simulink model "VAS_exec"  (Simulink 3.00)
undefined symbols (not defined in the file): BETA, PROJECT, REXYGEN, RPi, VAS, W1_owscfg
libraries: execlib x12

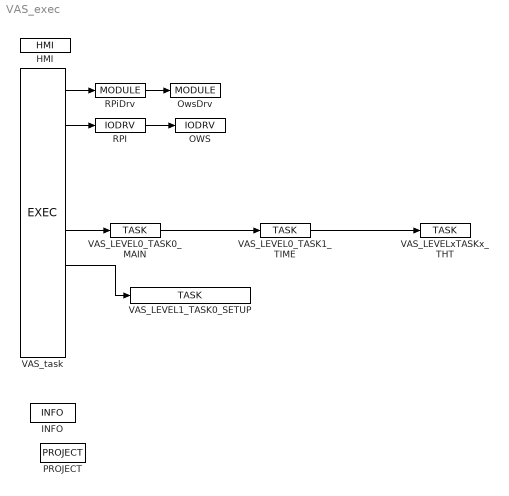
== system VAS_exec ==
  HMI : execlib/HMI  IncludeHMI=on  HmiDir=hmi  SourceDir=hmisrc  GenerateWebWatch=off  GenerateRexHMI=on  RedirectToHMI=on  Compression=on
  INFO : execlib/INFO  Title=VAS-REXYGEN-PROJECT-BETA  Author=Christopher Rothfeldt  Description=Vivarium Automation Server developed with REXYGEN by REX Controls  Customer=General
  OWS : execlib/IODRV  module=OwsDrv  classname=OwsDrv  cfgname=RPi-W1_owscfg.rio  factor=15  stack=10240  pri=3  timer=off
  OwsDrv : execlib/MODULE
  PROJECT : execlib/PROJECT  SourcesOnTarget=on
  RPI : execlib/IODRV  module=RPiDrv  classname=RPiDrv  factor=1  stack=10240  pri=3  timer=off
  RPiDrv : execlib/MODULE
  VAS_LEVEL0_TASK0_MAIN : execlib/TASK  factor=1  start=0  stop=1  stack=10240  MDLOPEN=on
  VAS_LEVEL0_TASK1_TIME : execlib/TASK  factor=1  start=1  stop=2  stack=10240  MDLOPEN=on
  VAS_LEVEL1_TASK0_SETUP : execlib/TASK  factor=1  start=0  stop=1  stack=10240  MDLOPEN=on
  VAS_LEVELxTASKx_THT : execlib/TASK  factor=1  start=2  stop=3  stack=10240  MDLOPEN=off
  "VAS_task " : execlib/EXEC  target=Generic target device  tick=0.05  ntick0=4  ntick1=10  ntick2=100  ntick3=1200  pri0=5  pri1=9  pri2=13  pri3=18
  wires:
  RPI/1 -> OWS/1
  RPiDrv/1 -> OwsDrv/1
  VAS_LEVEL0_TASK0_MAIN/1 -> VAS_LEVEL0_TASK1_TIME/1
  VAS_LEVEL0_TASK1_TIME/1 -> VAS_LEVELxTASKx_THT/1
  "VAS_task "/1 -> RPiDrv/1
  "VAS_task "/2 -> RPI/1
  "VAS_task "/5 -> VAS_LEVEL0_TASK0_MAIN/1
  "VAS_task "/6 -> VAS_LEVEL1_TASK0_SETUP/1
